simulink model "lr_motor_controller_design"  (R2017b)
settings: Solver=FixedStepAuto  StartTime=0.0  StopTime=10.0  FixedStep=Ts  RelTol=1e-3
values from neighbouring files (symbols this model uses):
  L_Kd = 0.52    [sim_params.m]
  L_Ke = 0.192    [l_motor_tf.m]    (also in sim_params.m)
  L_Ki = 40.0    (= 40)    [sim_params.m]
  L_Kp = 10.0    (= 10)    [sim_params.m]
  Max_V = Vbatt - Driver_Vdrop    (= 6.5)    [sim_params.m]
  Min_V = 3    [sim_params.m]
  R_Kd = 0.3    [sim_params.m]
  R_Ke = 0.226    [r_motor_tf.m]    (also in sim_params.m)
  R_Ki = 15.0    (= 15)    [sim_params.m]
  R_Kp = 5.5    [sim_params.m]
undefined symbols (not defined in the file or in its folder): alpha
libraries: simulink x2
settings Model: Creator=Devin  LastModifiedBy=Devin

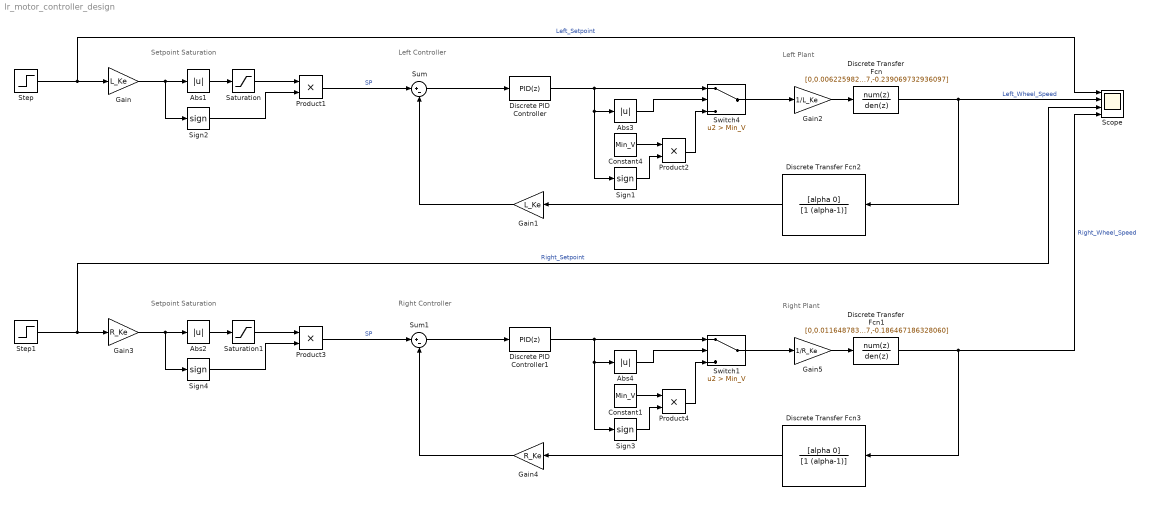
== system lr_motor_controller_design ==
  note: Setpoint Saturation
  note: Left Plant
  note: Left Controller
  note: Right Plant
  note: Setpoint Saturation
  note: Right Controller
  Abs{1..4} (4 alike) : Abs
  Constant1 : Constant  Value=Min_V
  Constant4 : Constant  Value=Min_V
  Discrete Transfer Fcn : DiscreteTransferFcn  Numerator=[0,0.00622598287442478,0.0173671875899039,0.00303706762075210]  Denominator=[1,-1.81883565031974,1.09137805901317,-0.239069732936097]
  Discrete Transfer Fcn1 : DiscreteTransferFcn  Numerator=[0,0.0116487831517155,0.0305659830219988,0.00501276447288935]  Denominator=[1,-1.68650783347506,0.914686419332717,-0.186467186328060]
  Discrete Transfer Fcn2 : DiscreteTransferFcn  Numerator=[alpha 0]  Denominator=[1 (alpha-1)]
  Discrete Transfer Fcn3 : DiscreteTransferFcn  Numerator=[alpha 0]  Denominator=[1 (alpha-1)]
  Discrete PID Controller : simulink/Continuous/PID Controller  Controller=PID  TimeDomain=Discrete-time  SampleTime=0.025  IntegratorMethod=Trapezoidal  FilterMethod=Forward Euler  Form=Parallel  UseFilter=off  ControllerParametersSource=internal  P=L_Kp  I=L_Ki  D=L_Kd  N=100  InitialConditionSource=internal  InitialConditionForIntegrator=0  InitialConditionForFilter=0  ExternalReset=none  LimitOutput=on  UpperSaturationLimit=Max_V  LowerSaturationLimit=-1* Min_V  LinearizeAsGain=off  AntiWindupMode=clamping  Kb=1  TrackingMode=off  Kt=1  PParamMin=[]  PParamMax=[]  IParamMin=[]  IParamMax=[]  DParamMin=[]  DParamMax=[]  NParamMin=[]  NParamMax=[]  KbParamMin=[]  KbParamMax=[]  KtParamMin=[]  KtParamMax=[]  POutMin=[]  POutMax=[]  IOutMin=[]  IOutMax=[]  DOutMin=[]  DOutMax=[]  NOutMin=[]  NOutMax=[]  KbOutMin=[]  KbOutMax=[]  KtOutMin=[]  KtOutMax=[]  IntegratorOutMin=[]  IntegratorOutMax=[]  FilterOutMin=[]  FilterOutMax=[]  SumOutMin=[]  SumOutMax=[]  SumI1OutMin=[]  SumI1OutMax=[]  SumI2OutMin=[]  SumI2OutMax=[]  SumI3OutMin=[]  SumI3OutMax=[]  SumDOutMin=[]  SumDOutMax=[]  SaturationOutMin=[]  SaturationOutMax=[]  IntegratorContinuousStateAttributes=''  IntegratorStateMustResolveToSignalObject=off  IntegratorRTWStateStorageClass=Auto  FilterContinuousStateAttributes=''  FilterStateMustResolveToSignalObject=off  FilterRTWStateStorageClass=Auto  DifferentiatorICPrevScaledInput=0  DifferentiatorOutMin=[]  DifferentiatorOutMax=[]  InitialConditionSetting=State (most efficient)  FilterDiffOutCoefMin=[]  FilterDiffOutCoefMax=[]  SumDenOutMin=[]  SumDenOutMax=[]  SumNumOutMin=[]  SumNumOutMax=[]  ReciprocalOutMin=[]  ReciprocalOutMax=[]  DivideOutMin=[]  DivideOutMax=[]  TunerSelectOption=Transfer Function Based (PID Tuner App)
  Discrete PID Controller1 : simulink/Continuous/PID Controller  Controller=PID  TimeDomain=Discrete-time  SampleTime=0.025  IntegratorMethod=Trapezoidal  FilterMethod=Forward Euler  Form=Parallel  UseFilter=off  ControllerParametersSource=internal  P=R_Kp  I=R_Ki  D=R_Kd  N=100  InitialConditionSource=internal  InitialConditionForIntegrator=0  InitialConditionForFilter=0  ExternalReset=none  LimitOutput=on  UpperSaturationLimit=Max_V  LowerSaturationLimit=-1* Min_V  LinearizeAsGain=off  AntiWindupMode=clamping  Kb=1  TrackingMode=off  Kt=1  PParamMin=[]  PParamMax=[]  IParamMin=[]  IParamMax=[]  DParamMin=[]  DParamMax=[]  NParamMin=[]  NParamMax=[]  KbParamMin=[]  KbParamMax=[]  KtParamMin=[]  KtParamMax=[]  POutMin=[]  POutMax=[]  IOutMin=[]  IOutMax=[]  DOutMin=[]  DOutMax=[]  NOutMin=[]  NOutMax=[]  KbOutMin=[]  KbOutMax=[]  KtOutMin=[]  KtOutMax=[]  IntegratorOutMin=[]  IntegratorOutMax=[]  FilterOutMin=[]  FilterOutMax=[]  SumOutMin=[]  SumOutMax=[]  SumI1OutMin=[]  SumI1OutMax=[]  SumI2OutMin=[]  SumI2OutMax=[]  SumI3OutMin=[]  SumI3OutMax=[]  SumDOutMin=[]  SumDOutMax=[]  SaturationOutMin=[]  SaturationOutMax=[]  IntegratorContinuousStateAttributes=''  IntegratorStateMustResolveToSignalObject=off  IntegratorRTWStateStorageClass=Auto  FilterContinuousStateAttributes=''  FilterStateMustResolveToSignalObject=off  FilterRTWStateStorageClass=Auto  DifferentiatorICPrevScaledInput=0  DifferentiatorOutMin=[]  DifferentiatorOutMax=[]  InitialConditionSetting=State (most efficient)  FilterDiffOutCoefMin=[]  FilterDiffOutCoefMax=[]  SumDenOutMin=[]  SumDenOutMax=[]  SumNumOutMin=[]  SumNumOutMax=[]  ReciprocalOutMin=[]  ReciprocalOutMax=[]  DivideOutMin=[]  DivideOutMax=[]  TunerSelectOption=Transfer Function Based (PID Tuner App)
  Gain : Gain  Gain=L_Ke
  Gain1 : Gain  Gain=L_Ke
  Gain2 : Gain  Gain=1/L_Ke
  Gain3 : Gain  Gain=R_Ke
  Gain4 : Gain  Gain=R_Ke
  Gain5 : Gain  Gain=1/R_Ke
  Product{1..4} (4 alike) : Product
  Saturation : Saturate  UpperLimit=Max_V  LowerLimit=Min_V
  Saturation1 : Saturate  UpperLimit=Max_V  LowerLimit=Min_V
  Scope : Scope  NumInputPorts=4
  Sign{1..4} (4 alike) : Signum
  Step : Step  After=18  SampleTime=0
  Step1 : Step  After=18  SampleTime=0
  Sum : Sum  Inputs=|+-
  Sum1 : Sum  Inputs=|+-
  Switch1 : Switch  Criteria=u2 > Threshold  Threshold=Min_V
  Switch4 : Switch  Criteria=u2 > Threshold  Threshold=Min_V
  wires:
  Discrete Transfer Fcn/1 -> Discrete Transfer Fcn2/1, Scope/2  "Left_Wheel_Speed"
  Sum/1 -> Discrete PID Controller/1
  Discrete PID Controller/1 -> Switch4/1, Sign1/1, Abs3/1
  Abs3/1 -> Switch4/2
  Constant4/1 -> Product2/1
  Sign1/1 -> Product2/2
  Product2/1 -> Switch4/3
  Switch4/1 -> Gain2/1
  Gain2/1 -> Discrete Transfer Fcn/1
  Product1/1 -> Sum/1  "SP"
  Step/1 -> Scope/1, Gain/1  "Left_Setpoint"
  Sign2/1 -> Product1/2
  Gain/1 -> Sign2/1, Abs1/1
  Gain1/1 -> Sum/2
  Abs1/1 -> Saturation/1
  Saturation/1 -> Product1/1
  Gain5/1 -> Discrete Transfer Fcn1/1
  Step1/1 -> Scope/3, Gain3/1  "Right_Setpoint"
  Sign4/1 -> Product3/2
  Sum1/1 -> Discrete PID Controller1/1
  Abs2/1 -> Saturation1/1
  Gain3/1 -> Sign4/1, Abs2/1
  Saturation1/1 -> Product3/1
  Constant1/1 -> Product4/1
  Abs4/1 -> Switch1/2
  Product4/1 -> Switch1/3
  Sign3/1 -> Product4/2
  Gain4/1 -> Sum1/2
  Discrete PID Controller1/1 -> Switch1/1, Sign3/1, Abs4/1
  Product3/1 -> Sum1/1  "SP"
  Discrete Transfer Fcn1/1 -> Discrete Transfer Fcn3/1, Scope/4  "Right_Wheel_Speed"
  Switch1/1 -> Gain5/1
  Discrete Transfer Fcn3/1 -> Gain4/1
  Discrete Transfer Fcn2/1 -> Gain1/1
